simulink library "RxTxFixedPointLibrary_noscopes"  (R2020a)
settings: Solver=VariableStepAuto  StartTime=0.0  StopTime=10.0  RelTol=1e-3
undefined symbols (not defined in the file): AGCBarkerSymbols, coeff, crcDecodeLag, CRCGeneratorLag, EQTrainingSymbols, j, K1, K2, numHeaderBits, numTrainingSamples, pLen, RadioSampleRate, samplesPerSymbol, VibertiTracebackLength, xPreambleSeq
libraries: simulink x32, dsphdlfiltering x20, hdlsllib x13, commseqgen3 x4, dspsigops x4, commdigbbndpm3 x3, commcrc2 x2, commcnvcod2 x2, $bdroot x1, dspstat3 x1, commfilt2 x1
(part 2 of 3)

== system RxTxFixedPointLibrary_noscopes/Receiver HDL/Viterbi Decode/Subsystem ==
  BypassVit : Inport
  bitsIn : Inport  Port=2
  Reset : Inport  Port=3
  Demux : Demux  Outputs=2
  Switch : Switch  Criteria=u2 > Threshold
  Terminator : Terminator
  Viterbi Decoder : commcnvcod2/Viterbi Decoder  trellis=poly2trellis(7, [171 133])  isPunctured=off  punctureVector=[1; 1; 0; 1; 0; 1]  erasures=off  dectype=Hard decision  nsdecb=4  runSigValErrCheck=off  tbdepth=VibertiTracebackLength  opmode=Continuous  reset=on  delayedResetAction=on  smWordLength=16  outDataType=boolean
      settings: SourceProductBaseCode=CM
  Viterbi Lag2 : Delay  DelayLength=VibertiTracebackLength
  bitsOut : Outport  VectorParamsAs1DForOutWhenUnconnected=off
  wires:
  Switch/1 -> bitsOut/1
  Viterbi Decoder/1 -> Switch/3
  Demux/1 -> Viterbi Lag2/1
  Reset/1 -> Viterbi Decoder/2
  bitsIn/1 -> Demux/1, Viterbi Decoder/1
  BypassVit/1 -> Switch/2
  Demux/2 -> Terminator/1
  Viterbi Lag2/1 -> Switch/1

== system RxTxFixedPointLibrary_noscopes/Transmitter HDL/Packet Generation/Create Header ==
  In1 : Inport
  Duplicate Header Bits : Concatenate
  Logical Operator : Logic  Operator=NOT  Inputs=1  AllPortsSameDT=off  OutDataTypeStr=boolean
  Out1 : Outport  VectorParamsAs1DForOutWhenUnconnected=off
  wires:
  In1/1 -> Duplicate Header Bits/1, Logical Operator/1
  Duplicate Header Bits/1 -> Out1/1
  Logical Operator/1 -> Duplicate Header Bits/2

== system RxTxFixedPointLibrary_noscopes/Transmitter HDL/Packet Generation/Payload ==
  data : Inport
  start : Inport  Port=2
  done : Inport  Port=3
  BypassEncode : Inport  Port=4
  Allow Reset : Delay  DelayLength=1
  Allow Reset1 : Delay  DelayLength=1
  Compensate For Reset : Delay  DelayLength=1
  Compensate For Reset1 : Delay  DelayLength=1
  Convolutional Encoder : Subsystem
  General CRC Generator HDL Optimized : commcrc2/General CRC Generator HDL Optimized  Polynomial=[1 0 0 0 0 0 1 0 0 1 1 0 0 0 0 0 1 0 0 0 1 1 1 0 1 1 0 1 1 0 1 1 1]  InitialState=0  DirectMethod=off  ReflectInput=off  ReflectCRCChecksum=off  FinalXORValue=0  SimulateUsing=Code generation
      settings: SourceProductBaseCode=CM
  HDL Scrambler : Subsystem  mask{poly=[1 1 0 1 0 1 0 1], init_state=[0 1 0 0 0 1 0]}
      mask prompts: poly "Polynomial"; init_state "Initial State"
  Latch : Subsystem
  Switch : Switch  Criteria=u2 > Threshold
  Trackback Delay : Delay  DelayLength=VibertiTracebackLength*2
  Viterbi Lag Stuffer : Subsystem
  bits : Outport  VectorParamsAs1DForOutWhenUnconnected=off
  end : Outport  Port=2  VectorParamsAs1DForOutWhenUnconnected=off
  valid : Outport  Port=3  VectorParamsAs1DForOutWhenUnconnected=off
  wires:
  General CRC Generator HDL Optimized/1 -> Allow Reset/1
  General CRC Generator HDL Optimized/4 -> Compensate For Reset1/1
  General CRC Generator HDL Optimized/2 -> Convolutional Encoder/3(Reset), HDL Scrambler/2(reset)
  Convolutional Encoder/1(bitsOut) -> bits/1
  Compensate For Reset/1 -> Viterbi Lag Stuffer/1(EOF), Trackback Delay/1
  General CRC Generator HDL Optimized/3 -> Compensate For Reset/1
  Compensate For Reset1/1 -> valid/1
  Trackback Delay/1 -> end/1
  Latch/1(Out1) -> General CRC Generator HDL Optimized/4
  done/1 -> Latch/2(In2), General CRC Generator HDL Optimized/3
  Switch/1 -> Convolutional Encoder/2(bitsIn)
  BypassEncode/1 -> Convolutional Encoder/1(BypassEncode)
  data/1 -> General CRC Generator HDL Optimized/1
  start/1 -> Allow Reset1/1
  Allow Reset1/1 -> Latch/1(In1), General CRC Generator HDL Optimized/2
  Allow Reset/1 -> HDL Scrambler/1(bitsIn)
  HDL Scrambler/1(bitsOut) -> Switch/3
  Viterbi Lag Stuffer/1(Bits) -> Switch/1
  Viterbi Lag Stuffer/2(Mode) -> Switch/2

== system RxTxFixedPointLibrary_noscopes/Transmitter HDL/Packet Generation/Preamble ==
  reset : Inport
  Barker Even : LookupNDDirect  NumberOfTableDimensions=1  Table=[PreambleBarkersBits(4:2:end),false(1,400)]  DiagnosticForOutOfRangeInput=Error  TableDataTypeStr=boolean
  Barker Odd : LookupNDDirect  NumberOfTableDimensions=1  Table=[PreambleBarkersBits(3:2:end-1),false(1,400)]  DiagnosticForOutOfRangeInput=Error  TableDataTypeStr=boolean
  Delay{,1..3} (4 alike) : Delay  DelayLength=1
  Enable at end of barker : simulink/Logic and Bit Operations/Compare To Constant  relop=<  const=pLen/2-1  OutDataTypeStr=boolean
  HDL Counter : hdlsllib/Sources/HDL Counter  CountType=Count limited  CountInit=0  CountStep=1  CountMax=pLen/2-2+400  CountFromType=Initial value  CountFrom=0  CountResetPort=on  CountLoadPort=off  CountEnbPort=off  CountDirPort=off  CountDataType=Unsigned  CountWordLen=16  CountFracLen=0  CountSampTime=1
  PN Sequence For EQ : commseqgen3/PN Sequence Generator  poly='z^5 + z^3 + z^1 + 1'  ini_sta=[1 1 1 0 0]  outBitMaskSource=Dialog parameter  shift=0  outVarSiz=off  maxOutSizeMode=Dialog parameter  maxOutSize=[10 1]  Ts=-1  sampPerFrame=1  reset=on  bitPackedOutputs=on  outDataType=double  numPackedBits=2  bitPackDataSigned=off  bitPackedOutDType=Smallest integer
  Reset When Barkers Are Done : simulink/Logic and Bit Operations/Compare To Constant  relop===  const=pLen/2-1  OutDataTypeStr=boolean
  Switch1 : Switch  Threshold=1
  Unpack1 : Subsystem
  Vector Concatenate1 : Concatenate
  Out1 : Outport  VectorParamsAs1DForOutWhenUnconnected=off
  wires:
  reset/1 -> HDL Counter/1
  Barker Odd/1 -> Vector Concatenate1/1
  Barker Even/1 -> Vector Concatenate1/2
  PN Sequence For EQ/1 -> Unpack1/1(In1)
  Switch1/1 -> Out1/1
  Reset When Barkers Are Done/1 -> PN Sequence For EQ/1
  HDL Counter/1 -> Delay/1
  Delay/1 -> Enable at end of barker/1, Reset When Barkers Are Done/1, Barker Even/1, Barker Odd/1
  Vector Concatenate1/1 -> Delay1/1
  Enable at end of barker/1 -> Delay2/1
  Unpack1/1(Out1) -> Delay3/1
  Delay1/1 -> Switch1/1
  Delay2/1 -> Switch1/2
  Delay3/1 -> Switch1/3

== system RxTxFixedPointLibrary_noscopes/Transmitter HDL/Packet Generation/Random Data ==
  In1 : Inport
  Random Data Gen1 : commseqgen3/PN Sequence Generator  poly='z^10 + z^7 + 1'  ini_sta=[0 0 1 0 0 1 0 0 1 1]  outBitMaskSource=Dialog parameter  shift=0  outVarSiz=off  maxOutSizeMode=Dialog parameter  maxOutSize=[10 1]  Ts=-1  sampPerFrame=1  reset=on  bitPackedOutputs=on  outDataType=double  numPackedBits=2  bitPackDataSigned=off  bitPackedOutDType=Smallest integer
  Unpack : Subsystem
  Out1 : Outport  VectorParamsAs1DForOutWhenUnconnected=off
  wires:
  In1/1 -> Random Data Gen1/1
  Unpack/1(Out1) -> Out1/1
  Random Data Gen1/1 -> Unpack/1(In1)

== system RxTxFixedPointLibrary_noscopes/Receiver HDL/CRC Check and DMA Pack/DMA Interface/Convert Payload Length To Bytes ==
  In1 : Inport
  Constant : Constant  Value=uint16(32-1)  SampleTime=-1
  Convert To Bytes From Bits : ArithShift  BitShiftNumber=3  BitShiftDirection=Right
  Convert To Uncoded : ArithShift  BitShiftNumber=1  BitShiftDirection=Right
  Data Type Conversion : DataTypeConversion  OutDataTypeStr=uint16
  Remove CRC Length : Sum  Inputs=+-  AccumDataTypeStr=uint16
  packetLengthOut : Outport  VectorParamsAs1DForOutWhenUnconnected=off
  wires:
  Data Type Conversion/1 -> packetLengthOut/1
  Constant/1 -> Remove CRC Length/2
  Convert To Bytes From Bits/1 -> Data Type Conversion/1
  Convert To Uncoded/1 -> Remove CRC Length/1
  Remove CRC Length/1 -> Convert To Bytes From Bits/1
  In1/1 -> Convert To Uncoded/1

== system RxTxFixedPointLibrary_noscopes/Receiver HDL/Frame Recover/Barker Locate/ABS1 ==
  In1 : Inport
  Add : Sum
  Complex to Real-Imag : ComplexToRealImag
  Product : Product  OutDataTypeStr=int16
  Product1 : Product  OutDataTypeStr=int16
  Out1 : Outport  VectorParamsAs1DForOutWhenUnconnected=off
  wires:
  Add/1 -> Out1/1
  Product1/1 -> Add/2
  Product/1 -> Add/1
  Complex to Real-Imag/1 -> Product/2, Product/1
  Complex to Real-Imag/2 -> Product1/1, Product1/2
  In1/1 -> Complex to Real-Imag/1

== system RxTxFixedPointLibrary_noscopes/Receiver HDL/Frame Recover/Barker Locate/ABS2 ==
  In1 : Inport
  Add : Sum  SaturateOnIntegerOverflow=on
  Complex to Real-Imag : ComplexToRealImag
  Product : Product  OutDataTypeStr=int16
  Product1 : Product  OutDataTypeStr=int16
  Out1 : Outport  VectorParamsAs1DForOutWhenUnconnected=off
  wires:
  Add/1 -> Out1/1
  Product1/1 -> Add/2
  Product/1 -> Add/1
  Complex to Real-Imag/1 -> Product/2, Product/1
  Complex to Real-Imag/2 -> Product1/1, Product1/2
  In1/1 -> Complex to Real-Imag/1

== system RxTxFixedPointLibrary_noscopes/Receiver HDL/Frame Recover/Barker Locate/HDL Opt Complex FIR ==
  In1 : Inport
  validIn : Inport  Port=2
  Add : Sum  AccumDataTypeStr=fixdt(1,16,0)
  Constant : Constant  Value=real(Taps)  OutDataTypeStr=fixdt(1,16)  SampleTime=-1
  Constant1 : Constant  Value=imag(Taps)  OutDataTypeStr=fixdt(1,16)  SampleTime=-1
  Discrete FIR Filter HDL Optimized : dsphdlfiltering/Discrete FIR Filter HDL Optimized  NumeratorSource=Input port (Parallel interface)  Numerator=real(Taps)  NumeratorPrototype=[]  FilterStructure=Direct form systolic  SerializationOption=Minimum number of cycles between valid input samples  NumberOfCycles=2  NumberOfMultipliers=2  SimulateUsing=Code generation  roundingMode=Floor  overflowMode=off  CoefficientsDataTypeStr=Inherit: Same word length as input  CoefficientsMin=[]  CoefficientsMax=[]  OutputDataTypeStr=fixdt(1,15,0)  OutputMin=[]  OutputMax=[]  ResetInputPort=off  HDLGlobalReset=off
      settings: SourceProductBaseCode=DS
  Discrete FIR Filter HDL Optimized1 : dsphdlfiltering/Discrete FIR Filter HDL Optimized  NumeratorSource=Input port (Parallel interface)  Numerator=imag(Taps)  NumeratorPrototype=[]  FilterStructure=Direct form systolic  SerializationOption=Minimum number of cycles between valid input samples  NumberOfCycles=2  NumberOfMultipliers=2  SimulateUsing=Code generation  roundingMode=Floor  overflowMode=off  CoefficientsDataTypeStr=Inherit: Same word length as input  CoefficientsMin=[]  CoefficientsMax=[]  OutputDataTypeStr=fixdt(1,15,0)  OutputMin=[]  OutputMax=[]  ResetInputPort=off  HDLGlobalReset=off
      settings: SourceProductBaseCode=DS
  Logical Operator : Logic  AllPortsSameDT=off  OutDataTypeStr=boolean
  Out1 : Outport  VectorParamsAs1DForOutWhenUnconnected=off
  validOut : Outport  Port=2  VectorParamsAs1DForOutWhenUnconnected=off
  wires:
  Constant1/1 -> Discrete FIR Filter HDL Optimized1/3
  Constant/1 -> Discrete FIR Filter HDL Optimized/3
  validIn/1 -> Discrete FIR Filter HDL Optimized/2, Discrete FIR Filter HDL Optimized1/2
  Discrete FIR Filter HDL Optimized1/1 -> Add/2
  Discrete FIR Filter HDL Optimized1/2 -> Logical Operator/2
  Discrete FIR Filter HDL Optimized/2 -> Logical Operator/1
  Logical Operator/1 -> validOut/1
  Add/1 -> Out1/1
  Discrete FIR Filter HDL Optimized/1 -> Add/1
  In1/1 -> Discrete FIR Filter HDL Optimized/1, Discrete FIR Filter HDL Optimized1/1

== system RxTxFixedPointLibrary_noscopes/Receiver HDL/Frame Recover/Barker Locate/Measure Phase Ambiguity ==
  data : Inport  OutDataTypeStr=int16
  trigger : Inport  Port=2
  validIn : Inport  Port=3
  Delay{,1..3} (4 alike) : Delay  DelayLength=1
  Find Max and Set Output Shift : Subsystem
  HDL Opt Complex FIR4 : Subsystem  mask{Taps=xPreambleSeq(end:-1:1).'}
  HDL Opt Complex FIR5 : Subsystem  mask{Taps=exp(-j*pi/2).*xPreambleSeq(end:-1:1).'}
  HDL Opt Complex FIR6 : Subsystem  mask{Taps=exp(-j*pi).*xPreambleSeq(end:-1:1).'}
  HDL Opt Complex FIR7 : Subsystem  mask{Taps=exp(-j*pi*3/2).*xPreambleSeq(end:-1:1).'}
  Logical Operator : Logic  Inputs=5  AllPortsSameDT=off  OutDataTypeStr=boolean
  Terminator : Terminator
  PA : Outport  InitialOutput=0  VectorParamsAs1DForOutWhenUnconnected=off
  wires:
  Logical Operator/1 -> Terminator/1
  Delay3/1 -> Find Max and Set Output Shift/1(In1)
  Delay2/1 -> Find Max and Set Output Shift/2(In2)
  Delay1/1 -> Find Max and Set Output Shift/3(In4)
  Delay/1 -> Find Max and Set Output Shift/4(In5)
  trigger/1 -> Logical Operator/5, Find Max and Set Output Shift/Enable
  HDL Opt Complex FIR7/2(validOut) -> Logical Operator/4
  HDL Opt Complex FIR6/2(validOut) -> Logical Operator/3
  HDL Opt Complex FIR5/2(validOut) -> Logical Operator/2
  HDL Opt Complex FIR4/2(validOut) -> Logical Operator/1
  validIn/1 -> HDL Opt Complex FIR6/2(validIn), HDL Opt Complex FIR7/2(validIn), HDL Opt Complex FIR5/2(validIn), HDL Opt Complex FIR4/2(validIn)
  Find Max and Set Output Shift/1(Out1) -> PA/1
  HDL Opt Complex FIR7/1(Out1) -> Delay/1
  HDL Opt Complex FIR6/1(Out1) -> Delay1/1
  HDL Opt Complex FIR5/1(Out1) -> Delay2/1
  HDL Opt Complex FIR4/1(Out1) -> Delay3/1
  data/1 -> HDL Opt Complex FIR6/1(In1), HDL Opt Complex FIR7/1(In1), HDL Opt Complex FIR5/1(In1), HDL Opt Complex FIR4/1(In1)

== system RxTxFixedPointLibrary_noscopes/Receiver HDL/Frame Recover/Equalization and Demodulation/DFE ==
  note: Generate training sequence when barker is found
  note: refTap=0 to disableEQ
  Trigger : Inport  PortDimensions=1
  data : Inport  Port=2  PortDimensions=1
      settings: SignalType=complex
  EQmu : Inport  Port=3
  eqBypass : Inport  Port=4
  DFE : Subsystem  mask{numFTaps=5, numBTaps=3, mu=0.01, refTap=2}
      mask prompts: numFTaps "Num Forward Taps"; numBTaps "Num Backward Taps"; mu "Step Size"; refTap "Reference Tap"
  Delay data so DFE can reset : Delay  DelayLength=1
  Delay ref so DFE can reset : Delay  DelayLength=1
  Equalizer : MATLAB Function  Commented=on  TreatAsAtomicUnit=on
  PN Sequence Generator : commseqgen3/PN Sequence Generator  poly='z^5 + z^3 + z^1 + 1'  ini_sta=[1 1 1 0 0]  outBitMaskSource=Dialog parameter  shift=0  outVarSiz=off  maxOutSizeMode=Dialog parameter  maxOutSize=[10 1]  Ts=-1  sampPerFrame=1  reset=on  bitPackedOutputs=on  outDataType=Smallest unsigned integer  numPackedBits=2  bitPackDataSigned=off  bitPackedOutDType=Smallest integer
  Packeted To Unpacked : Subsystem
  QPSK Modulator Baseband : commdigbbndpm3/QPSK Modulator Baseband  InType=Bit  Enc=Binary  Ph=pi/4  outDtype=Fixed-point  outWordLen=16  outUDDataType=sfix(16)  outFracLenMode=User-defined  outFracLen=15  outDataTypeStr=fixdt(1,16,15)  outLastDataTypeStr=fixdt(1,16,15)
  Terminator1 : Terminator
  dataEQed : Outport  VectorParamsAs1DForOutWhenUnconnected=off
  start : Outport  Port=2  VectorParamsAs1DForOutWhenUnconnected=off
  wires:
  EQmu/1 -> DFE/4(EQmu)
  Delay ref so DFE can reset/1 -> DFE/3(training)
  Delay data so DFE can reset/1 -> DFE/2(dataIn)
  DFE/1(eqOut) -> dataEQed/1
  DFE/2(err) -> Terminator1/1
  Trigger/1 -> PN Sequence Generator/1, DFE/1(reset)
  DFE/3(start) -> start/1
  QPSK Modulator Baseband/1 -> Delay ref so DFE can reset/1
  Packeted To Unpacked/1(Out1) -> QPSK Modulator Baseband/1
  PN Sequence Generator/1 -> Packeted To Unpacked/1(In1)
  data/1 -> Delay data so DFE can reset/1
  eqBypass/1 -> DFE/5(eqBypass)

== system RxTxFixedPointLibrary_noscopes/Receiver HDL/Frame Recover/Frequency Recovery/Lock Detector ==
  ped : Inport
  Compare To Constant : simulink/Logic and Bit Operations/Compare To Constant  relop=<=  const=Threshold*WindowLength  OutDataTypeStr=boolean
  MATLAB Function : MATLAB Function  TreatAsAtomicUnit=on
  Pipeline Delay{,1..3} (4 alike) : Delay  DelayLength=1
  Sum of Elements : Sum  Inputs=+
  Tapped Delay : simulink/Discrete/Tapped Delay  vinit=0.0  samptime=-1  NumDelays=WindowLength  DelayOrder=Oldest  includeCurrent=off
  lock : Outport  VectorParamsAs1DForOutWhenUnconnected=off
  wires:
  ped/1 -> Pipeline Delay/1
  Tapped Delay/1 -> Pipeline Delay2/1
  Sum of Elements/1 -> Pipeline Delay3/1
  Compare To Constant/1 -> lock/1
  MATLAB Function/1(y) -> Pipeline Delay1/1
  Pipeline Delay/1 -> MATLAB Function/1(u)
  Pipeline Delay1/1 -> Tapped Delay/1
  Pipeline Delay2/1 -> Sum of Elements/1
  Pipeline Delay3/1 -> Compare To Constant/1

== system RxTxFixedPointLibrary_noscopes/Receiver HDL/Frame Recover/Frequency Recovery/Loop Filter ==
  note: Proportional-plus-Integrator Loop Filter,
      | Infinite DC Response to guarantee convergence
  note: This inflation is necessary
  e : Inport
  Add1 : Sum  RndMeth=Nearest  OutDataTypeStr=Inherit: Same as first input
  Add2 : Sum  OutDataTypeStr=Inherit: Same as first input
  Data Type Conversion : DataTypeConversion  OutDataTypeStr=fixdt(1,25,20)
  Delay : Delay  DelayLength=1
  Delay3 : Delay  DelayLength=1
  Delay4 : Delay  DelayLength=1
  K1 : Gain  Gain=K2  OutDataTypeStr=Inherit: Same as input
  K2 : Gain  Gain=K1  OutDataTypeStr=Inherit: Same as input
  Sum2 : Sum  OutDataTypeStr=Inherit: Same as first input
  v : Outport  VectorParamsAs1DForOutWhenUnconnected=off
  wires:
  Data Type Conversion/1 -> v/1
  Add2/1 -> Data Type Conversion/1, Delay4/1
  Delay4/1 -> Add2/2
  Delay3/1 -> Add2/1
  Sum2/1 -> Delay3/1
  Delay/1 -> Add1/1
  K2/1 -> Add1/2, Delay/1
  e/1 -> K1/1, K2/1
  Add1/1 -> Sum2/2
  K1/1 -> Sum2/1

== system RxTxFixedPointLibrary_noscopes/Receiver HDL/Frame Recover/Frequency Recovery/Loop Filter Configurable ==
  note: Proportional-plus-Integrator Loop Filter,
      | Infinite DC Response to guarantee convergence
  note: This inflation is necessary
  e : Inport
  LoopBW : Inport  Port=2
  Add1 : Sum  RndMeth=Nearest  OutDataTypeStr=Inherit: Same as first input
  Add2 : Sum  OutDataTypeStr=Inherit: Same as first input
  Data Type Conversion : DataTypeConversion  OutDataTypeStr=fixdt(1,25,20)
  Delay : Delay  DelayLength=1
  Delay3 : Delay  DelayLength=1
  Delay4 : Delay  DelayLength=1
  Direct Lookup Table (n-D) : LookupNDDirect  NumberOfTableDimensions=1  Table=K1  DiagnosticForOutOfRangeInput=Error
  Direct Lookup Table (n-D)1 : LookupNDDirect  NumberOfTableDimensions=1  Table=K2  DiagnosticForOutOfRangeInput=Error
  Product : Product  OutDataTypeStr=Inherit: Same as first input
  Product1 : Product  OutDataTypeStr=Inherit: Same as first input
  Sum2 : Sum  OutDataTypeStr=Inherit: Same as first input
  v : Outport  VectorParamsAs1DForOutWhenUnconnected=off
  wires:
  LoopBW/1 -> Direct Lookup Table (n-D)1/1, Direct Lookup Table (n-D)/1
  Direct Lookup Table (n-D)1/1 -> Product1/2
  Direct Lookup Table (n-D)/1 -> Product/2
  Data Type Conversion/1 -> v/1
  Add2/1 -> Data Type Conversion/1, Delay4/1
  Delay4/1 -> Add2/2
  Delay3/1 -> Add2/1
  Sum2/1 -> Delay3/1
  Delay/1 -> Add1/1
  Product1/1 -> Add1/2, Delay/1
  e/1 -> Product/1, Product1/1
  Add1/1 -> Sum2/2
  Product/1 -> Sum2/1

== system RxTxFixedPointLibrary_noscopes/Receiver HDL/Frame Recover/Frequency Recovery/Phase Shift FP ==
  note: Sign Comes from original
      | loop filter design
  In1 : Inport
  Phi : Inport  Port=2
  Cosine HDL Optimized : hdlsllib/Lookup Tables/Cosine HDL Optimized  OutputFormula=exp(j*2*pi*u)  NumDataPoints=256  TableDataTypeStr=fixdt(0,31,20)  SimulateLUTROMDelay=off
      settings: SourceProductBaseCode=SL
  Gain : Gain  Gain=-1/(2*pi)  ParamDataTypeStr=fixdt(1,25,20)  OutDataTypeStr=fixdt(1,16,12)  SaturateOnIntegerOverflow=on
  Product : Product  OutDataTypeStr=fixdt(1,16,13)  SaturateOnIntegerOverflow=on
  Out1 : Outport  VectorParamsAs1DForOutWhenUnconnected=off
  wires:
  Gain/1 -> Cosine HDL Optimized/1
  Phi/1 -> Gain/1
  In1/1 -> Product/1
  Cosine HDL Optimized/1 -> Product/2
  Product/1 -> Out1/1

== system RxTxFixedPointLibrary_noscopes/Receiver HDL/Frame Recover/Gardner Timing Recovery/Gardner TED Blocks ==
  note: This is for QPSK and 4 SamplesPerSymbol ONLY
  note: An input of 4 should not
      | happen unless the input is all zeros
  data : Inport
  strobe : Inport  Port=2
  Add : Sum  OutDataTypeStr=fixdt(1,16,15)
  Check Only Strobe Condition : simulink/Logic and Bit Operations/Compare To Constant  relop===  const=uint8(1)  OutDataTypeStr=boolean
  Complex to Real-Imag : ComplexToRealImag
  Constant : Constant  Value=0  OutDataTypeStr=Inherit: Inherit via back propagation  SampleTime=-1
  Display : Display
  Imag Error : Subsystem
  Logical Operator : Logic  AllPortsSameDT=off  OutDataTypeStr=boolean
  Map [0,1,2,3,4] to [0,1,2,2,2] : LookupNDDirect  NumberOfTableDimensions=1  Table=[0 1 2 2 2]  DiagnosticForOutOfRangeInput=Error  TableDataTypeStr=uint8
  Real Error : Subsystem
  Strobe Buffer1 : simulink/Discrete/Tapped Delay  vinit=0.0  samptime=-1  NumDelays=samplesPerSymbol-1  DelayOrder=Oldest  includeCurrent=on
  Sum of Elements1 : Sum  Inputs=+  OutDataTypeStr=int8
  Switch : Switch  Criteria=u2 ~= 0  SaturateOnIntegerOverflow=on
  e : Outport  VectorParamsAs1DForOutWhenUnconnected=off
  wires:
  Logical Operator/1 -> Switch/2
  Add/1 -> Switch/1
  Imag Error/1(Out1) -> Add/2
  Real Error/1(Out1) -> Add/1
  Strobe Buffer1/1 -> Sum of Elements1/1
  Map [0,1,2,3,4] to [0,1,2,2,2]/1 -> Real Error/2(strobe sum), Imag Error/2(strobe sum)
  data/1 -> Complex to Real-Imag/1
  Complex to Real-Imag/1 -> Real Error/1(data)
  Constant/1 -> Switch/3
  Check Only Strobe Condition/1 -> Logical Operator/1
  Sum of Elements1/1 -> Map [0,1,2,3,4] to [0,1,2,2,2]/1, Check Only Strobe Condition/1, Display/1
  Complex to Real-Imag/2 -> Imag Error/1(data)
  strobe/1 -> Logical Operator/2, Strobe Buffer1/1
  Switch/1 -> e/1

== system RxTxFixedPointLibrary_noscopes/Receiver HDL/Frame Recover/Gardner Timing Recovery/InterpControl_Blocks1 ==
  note: Mu is always positive
  note: e<<1/SPS
  e : Inport
  1/SPS1 : Constant  Value=fi(1/samplesPerSymbol,0,2,2)  OutDataTypeStr=fixdt(0,2,2)  SampleTime=-1
  Add1 : Sum  OutDataTypeStr=fixdt(0,16,16)
  Calculate New mu : Subsystem
  Display{,1..3} (4 alike) : Display
  Mod 1 : Subsystem
  NCOCounter State : Delay  DelayLength=1  InitialCondition=0
  Subtract1 : Sum  Inputs=-+  OutDataTypeStr=Inherit: Same as first input
  Update mu on strobe : Switch  Criteria=u2 > Threshold
  saved mu : Delay  DelayLength=1
  strobe == W>NCOCounter : RelationalOperator  Operator=>  OutDataTypeStr=boolean  RndMeth=Nearest
  strobe : Outport  VectorParamsAs1DForOutWhenUnconnected=off
  mu : Outport  Port=2  VectorParamsAs1DForOutWhenUnconnected=off
  wires:
  Add1/1 -> Subtract1/1, Display2/1, strobe == W>NCOCounter/1, Calculate New mu/1(W)
  1/SPS1/1 -> Add1/2
  Mod 1/1(Out1) -> NCOCounter State/1
  Subtract1/1 -> Mod 1/1(In1)
  NCOCounter State/1 -> Calculate New mu/2(NCOCounter), strobe == W>NCOCounter/2, Display1/1, Subtract1/2
  e/1 -> Add1/1
  Calculate New mu/1(mu) -> Update mu on strobe/1, Display/1
  saved mu/1 -> Update mu on strobe/3
  Update mu on strobe/1 -> saved mu/1, mu/1, Display3/1
  strobe == W>NCOCounter/1 -> strobe/1, Update mu on strobe/2

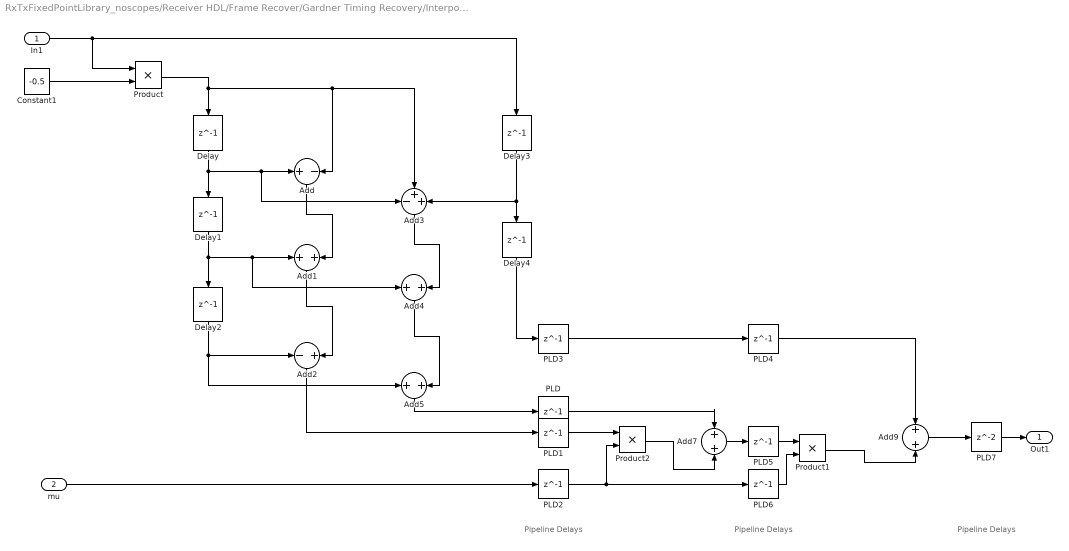
== system RxTxFixedPointLibrary_noscopes/Receiver HDL/Frame Recover/Gardner Timing Recovery/Interpolator ==
  note: Pipeline Delays
  note: Pipeline Delays
  note: Pipeline Delays
  In1 : Inport
  mu : Inport  Port=2
  Add : Sum  Inputs=+-  OutDataTypeStr=Inherit: Same as first input
  Add{1,4..5,7} (4 alike) : Sum
  Add2 : Sum  Inputs=-+
  Add3 : Sum  Inputs=-++
  Add9 : Sum  OutDataTypeStr=fixdt(1,16,10)
  Constant1 : Constant  Value=-0.5  OutDataTypeStr=fixdt(1,2,2)  SampleTime=-1
  Delay{,1..4} (5 alike) : Delay  DelayLength=1
  PLD{,1..6} (7 alike) : Delay  DelayLength=1
  PLD7 : Delay
  Product : Product  OutDataTypeStr=fixdt(1,16,14)
  Product1 : Product
  Product2 : Product  OutDataTypeStr=fixdt(1,16,10)
  Out1 : Outport  VectorParamsAs1DForOutWhenUnconnected=off
  wires:
  PLD7/1 -> Out1/1
  PLD6/1 -> Product1/2
  PLD5/1 -> Product1/1
  PLD4/1 -> Add9/1
  PLD3/1 -> PLD4/1
  PLD2/1 -> PLD6/1, Product2/2
  PLD1/1 -> Product2/1
  PLD/1 -> Add7/1
  Constant1/1 -> Product/2
  Product1/1 -> Add9/2
  Add7/1 -> PLD5/1
  Delay4/1 -> PLD3/1
  Delay3/1 -> Add3/3, Delay4/1
  Add9/1 -> PLD7/1
  Product2/1 -> Add7/2
  Add5/1 -> PLD/1
  mu/1 -> PLD2/1
  Add2/1 -> PLD1/1
  Add4/1 -> Add5/2
  Add3/1 -> Add4/2
  Add1/1 -> Add2/2
  Delay2/1 -> Add2/1, Add5/1
  Add/1 -> Add1/2
  Delay1/1 -> Delay2/1, Add1/1, Add4/1
  Delay/1 -> Delay1/1, Add/1, Add3/1
  Product/1 -> Delay/1, Add/2, Add3/2
  In1/1 -> Product/1, Delay3/1

== system RxTxFixedPointLibrary_noscopes/Receiver HDL/Frame Recover/Gardner Timing Recovery/LoopFilter1 ==
  e : Inport
  Delay1 : Delay  DelayLength=1
  Delay2 : Delay  DelayLength=1
  Proportional Gain : Gain  Gain=fi(ProportionalGain,1,16,15)  OutDataTypeStr=fixdt(1,16,24)
  v : Outport  VectorParamsAs1DForOutWhenUnconnected=off
  wires:
  Delay1/1 -> v/1
  Delay2/1 -> Proportional Gain/1
  Proportional Gain/1 -> Delay1/1
  e/1 -> Delay2/1

== system RxTxFixedPointLibrary_noscopes/Receiver HDL/Frame Recover/Gardner Timing Recovery/TED Lock Detector ==
  ted : Inport
  Compare To Constant : simulink/Logic and Bit Operations/Compare To Constant  relop=<=  const=Threshold*WindowLength  OutDataTypeStr=boolean
  MATLAB Function : MATLAB Function  TreatAsAtomicUnit=on
  Pipeline Delay{,1..3} (4 alike) : Delay  DelayLength=1
  Sum of Elements : Sum  Inputs=+
  Tapped Delay : simulink/Discrete/Tapped Delay  vinit=0.0  samptime=-1  NumDelays=WindowLength  DelayOrder=Oldest  includeCurrent=off
  lock : Outport  VectorParamsAs1DForOutWhenUnconnected=off
  wires:
  ted/1 -> Pipeline Delay/1
  Tapped Delay/1 -> Pipeline Delay1/1
  Sum of Elements/1 -> Pipeline Delay3/1
  Compare To Constant/1 -> lock/1
  MATLAB Function/1(y) -> Pipeline Delay2/1
  Pipeline Delay/1 -> MATLAB Function/1(u)
  Pipeline Delay1/1 -> Sum of Elements/1
  Pipeline Delay2/1 -> Tapped Delay/1
  Pipeline Delay3/1 -> Compare To Constant/1

== system RxTxFixedPointLibrary_noscopes/Receiver HDL/Frame Recover/Manage Error Signals/Debug: Header Check ==
  <status> : Inport
  <s1> : Inport  Port=2
  <s2> : Inport  Port=3
  Enable : EnablePort
  DEBUG: Header : MATLAB Function  TreatAsAtomicUnit=on
  wires:
  <s1>/1 -> DEBUG: Header/2(h1)
  <status>/1 -> DEBUG: Header/1(status)
  <s2>/1 -> DEBUG: Header/3(h2)

== system RxTxFixedPointLibrary_noscopes/Receiver HDL/Viterbi Decode/Buffer Frame/Check Packet Size ==
  In1 : Inport
  In2 : Inport  Port=2
  In3 : Inport  Port=3
  Compare To Zero : simulink/Logic and Bit Operations/Compare To Zero  relop=~=  OutDataTypeStr=boolean
  HDL Counter1 : hdlsllib/Sources/HDL Counter  CountType=Count limited  CountInit=0  CountStep=1  CountMax=2^16-1  CountFromType=Initial value  CountFrom=0  CountResetPort=off  CountLoadPort=off  CountEnbPort=on  CountDirPort=off  CountDataType=Unsigned  CountWordLen=16  CountFracLen=0  CountSampTime=1
  Logical Operator1 : Logic  AllPortsSameDT=off  OutDataTypeStr=boolean
  Pipeline Delay{,1..3} (4 alike) : Delay  DelayLength=1
  Subtract1 : Sum  Inputs=+-
  Out1 : Outport  VectorParamsAs1DForOutWhenUnconnected=off
  wires:
  Pipeline Delay3/1 -> Out1/1
  Pipeline Delay2/1 -> Logical Operator1/2
  Pipeline Delay1/1 -> Subtract1/2
  Pipeline Delay/1 -> Subtract1/1
  In3/1 -> Pipeline Delay2/1
  HDL Counter1/1 -> Pipeline Delay3/1
  In1/1 -> Pipeline Delay/1
  In2/1 -> Pipeline Delay1/1
  Logical Operator1/1 -> HDL Counter1/1
  Compare To Zero/1 -> Logical Operator1/1
  Subtract1/1 -> Compare To Zero/1

== system RxTxFixedPointLibrary_noscopes/Receiver HDL/Viterbi Decode/Buffer Frame/FIFO ==
  dataIn : Inport
  Push : Inport  Port=2
  Pop : Inport  Port=3
  Demux : Demux  Outputs=2
  HDL FIFO3 : hdlsllib/HDL RAMs/HDL FIFO  fifo_size=2^16  mode=Classic  ratio=1  push_msg=Warning  pop_msg=Warning  show_empty=off  show_full=off  show_num=on  LabelModeActiveChoice_Mode=Classic
      settings: SourceProductBaseCode=SL
  HDL FIFO4 : hdlsllib/HDL RAMs/HDL FIFO  fifo_size=2^16  mode=Classic  ratio=1  push_msg=Warning  pop_msg=Warning  show_empty=off  show_full=off  show_num=off  LabelModeActiveChoice_Mode=Classic
      settings: SourceProductBaseCode=SL
  Mux : Mux  Inputs=2
  dataOut : Outport  VectorParamsAs1DForOutWhenUnconnected=off
  Count : Outport  Port=2  VectorParamsAs1DForOutWhenUnconnected=off
  wires:
  HDL FIFO3/2 -> Count/1
  HDL FIFO4/1 -> Mux/2
  Mux/1 -> dataOut/1
  HDL FIFO3/1 -> Mux/1
  Demux/2 -> HDL FIFO4/1
  Demux/1 -> HDL FIFO3/1
  dataIn/1 -> Demux/1
  Push/1 -> HDL FIFO3/2, HDL FIFO4/2
  Pop/1 -> HDL FIFO3/3, HDL FIFO4/3

== system RxTxFixedPointLibrary_noscopes/Receiver HDL/Viterbi Decode/Buffer Frame/Latch ==
  In1 : Inport
  In2 : Inport  Port=2
  Delay2 : Delay  DelayLength=1
  Switch : Switch  Criteria=u2 > Threshold  OutDataTypeStr=fixdt(0,17,0)
  Out1 : Outport  VectorParamsAs1DForOutWhenUnconnected=off
  wires:
  Switch/1 -> Delay2/1, Out1/1
  Delay2/1 -> Switch/3
  In1/1 -> Switch/1
  In2/1 -> Switch/2

== system RxTxFixedPointLibrary_noscopes/Receiver HDL/Viterbi Decode/Descrambler1/Resetabled Tapped Delay ==
  In1 : Inport
  Reset : ResetPort  DisableCoverage=on  ResetTriggerType=level hold
  State Control : StateControl  StateControl=Synchronous
  Tapped Delay : simulink/Discrete/Tapped Delay  vinit=initstate(1:end)  samptime=-1  NumDelays=length(initstate)  DelayOrder=Oldest  includeCurrent=off
  Out1 : Outport  VectorParamsAs1DForOutWhenUnconnected=off
  wires:
  In1/1 -> Tapped Delay/1
  Tapped Delay/1 -> Out1/1

== system RxTxFixedPointLibrary_noscopes/Transmitter HDL/Packet Generation/Payload/Convolutional Encoder ==
  BypassEncode : Inport
  bitsIn : Inport  Port=2
  Reset : Inport  Port=3
  Convolutional Encoder : commcnvcod2/Convolutional Encoder  trellis=poly2trellis(7, [171 133])  opMode=Reset on nonzero input via port  DelayedResetAction=on  hasIniStPort=off  hasFinStPort=off  usePuncVector=off  punctureVector=[1; 1; 0; 1; 0; 1]  reset=Unused parameter value
      settings: SourceProductBaseCode=CM
  Mux : Mux  Inputs=2
  Signal Specification : SignalSpecification  Dimensions=2
  Switch1 : Switch  Criteria=u2 > Threshold
  bitsOut : Outport  VectorParamsAs1DForOutWhenUnconnected=off
  wires:
  bitsIn/1 -> Mux/2, Mux/1, Convolutional Encoder/1
  Mux/1 -> Switch1/1
  Reset/1 -> Convolutional Encoder/2
  BypassEncode/1 -> Switch1/2
  Switch1/1 -> bitsOut/1
  Convolutional Encoder/1 -> Signal Specification/1
  Signal Specification/1 -> Switch1/3

== system RxTxFixedPointLibrary_noscopes/Transmitter HDL/Packet Generation/Payload/HDL Scrambler ==
  bitsIn : Inport
  reset : Inport  Port=2
  Resettable Synchronous Subsystem : Subsystem  TreatAsAtomicUnit=on
  Selector2 : Selector  IndexOptions=Index vector (dialog)  Indices=find(poly(2:end))  OutputSizes=1
  state_xor5 : Logic  Operator=XOR  Inputs=1  IconShape=distinctive  AllPortsSameDT=off  OutDataTypeStr=boolean
  state_xor6 : Logic  Operator=XOR  IconShape=distinctive  AllPortsSameDT=off  OutDataTypeStr=boolean
  bitsOut : Outport  VectorParamsAs1DForOutWhenUnconnected=off
  wires:
  reset/1 -> Resettable Synchronous Subsystem/Reset
  Selector2/1 -> state_xor5/1
  state_xor5/1 -> state_xor6/1
  bitsIn/1 -> state_xor6/2
  Resettable Synchronous Subsystem/1(Out1) -> Selector2/1
  state_xor6/1 -> Resettable Synchronous Subsystem/1(In1), bitsOut/1

== system RxTxFixedPointLibrary_noscopes/Transmitter HDL/Packet Generation/Payload/Latch ==
  In1 : Inport
  In2 : Inport  Port=2
  Logical Operator : Logic  Operator=OR  Inputs=3  AllPortsSameDT=off  OutDataTypeStr=boolean
  MATLAB Function3 : MATLAB Function  TreatAsAtomicUnit=on
  Out1 : Outport  VectorParamsAs1DForOutWhenUnconnected=off
  wires:
  In2/1 -> Logical Operator/3, MATLAB Function3/2(done)
  In1/1 -> Logical Operator/1, MATLAB Function3/1(start)
  MATLAB Function3/1(enable) -> Logical Operator/2
  Logical Operator/1 -> Out1/1

== system RxTxFixedPointLibrary_noscopes/Transmitter HDL/Packet Generation/Payload/Viterbi Lag Stuffer ==
  EOF : Inport
  Compensate For Data2 : Delay  DelayLength=1
  MATLAB Function : MATLAB Function  TreatAsAtomicUnit=on
  Random Data Gen1 : commseqgen3/PN Sequence Generator  poly='z^10 + z^7 + 1'  ini_sta=[0 0 1 0 0 1 0 0 1 1]  outBitMaskSource=Dialog parameter  shift=0  outVarSiz=off  maxOutSizeMode=Dialog parameter  maxOutSize=[10 1]  Ts=-1  sampPerFrame=1  reset=on  bitPackedOutputs=on  outDataType=double  numPackedBits=1  bitPackDataSigned=off  bitPackedOutDType=Smallest integer
  Bits : Outport  VectorParamsAs1DForOutWhenUnconnected=off
  Mode : Outport  Port=2  VectorParamsAs1DForOutWhenUnconnected=off
  wires:
  MATLAB Function/2(mode) -> Mode/1
  MATLAB Function/1(reset) -> Random Data Gen1/1
  Random Data Gen1/1 -> Bits/1
  Compensate For Data2/1 -> MATLAB Function/1(enable)
  EOF/1 -> Compensate For Data2/1

== system RxTxFixedPointLibrary_noscopes/Transmitter HDL/Packet Generation/Preamble/Unpack1 ==
  In1 : Inport
  Data Type Conversion : DataTypeConversion  OutDataTypeStr=boolean
  Extract Bits : simulink/Logic and Bit Operations/Extract Bits  bitsToExtract=Range of bits  numBits=8  bitIdxRange=[1]  outScalingMode=Treat bit field as an integer
  Extract Bits1 : simulink/Logic and Bit Operations/Extract Bits  bitsToExtract=Range of bits  numBits=8  bitIdxRange=[0]  outScalingMode=Treat bit field as an integer
  Vector Concatenate : Concatenate
  Out1 : Outport  VectorParamsAs1DForOutWhenUnconnected=off
  wires:
  In1/1 -> Extract Bits1/1, Extract Bits/1
  Extract Bits/1 -> Vector Concatenate/1
  Extract Bits1/1 -> Vector Concatenate/2
  Vector Concatenate/1 -> Data Type Conversion/1
  Data Type Conversion/1 -> Out1/1

== system RxTxFixedPointLibrary_noscopes/Transmitter HDL/Packet Generation/Random Data/Unpack ==
  In1 : Inport
  Data Type Conversion : DataTypeConversion  OutDataTypeStr=boolean
  Extract Bits : simulink/Logic and Bit Operations/Extract Bits  bitsToExtract=Range of bits  numBits=8  bitIdxRange=[0]  outScalingMode=Treat bit field as an integer
  Extract Bits1 : simulink/Logic and Bit Operations/Extract Bits  bitsToExtract=Range of bits  numBits=8  bitIdxRange=[1]  outScalingMode=Treat bit field as an integer
  Vector Concatenate : Concatenate
  Out1 : Outport  VectorParamsAs1DForOutWhenUnconnected=off
  wires:
  In1/1 -> Extract Bits1/1, Extract Bits/1
  Extract Bits/1 -> Vector Concatenate/1
  Extract Bits1/1 -> Vector Concatenate/2
  Vector Concatenate/1 -> Data Type Conversion/1
  Data Type Conversion/1 -> Out1/1

== system RxTxFixedPointLibrary_noscopes/Receiver HDL/Frame Recover/Barker Locate/Measure Phase Ambiguity/Find Max and Set Output Shift ==
  In1 : Inport
  In2 : Inport  Port=2
  In4 : Inport  Port=3
  In5 : Inport  Port=4
  Enable : EnablePort
  Complex to Real-Imag{,1..3} (4 alike) : ComplexToRealImag  Output=Imag
  Direct Lookup Table (n-D)1 : LookupNDDirect  Commented=on  NumberOfTableDimensions=1  Table=-1i.*ones(1,4)  DiagnosticForOutOfRangeInput=Error  TableDataTypeStr=fixdt(1,16,13)
  Direct Lookup Table (n-D)2 : LookupNDDirect  NumberOfTableDimensions=1  Table=exp(-(0:pi/2:(pi*3/2)) .* 1i).'  DiagnosticForOutOfRangeInput=Error  TableDataTypeStr=fixdt(1,16,13)
  Maximum : dspstat3/Maximum  operation=maximum  fcn=Index  indexBase=Zero  operateOver=Each column  Dimension=1  InputProcessing=Columns as channels (frame based)  reset=None  roiEnable=off  roiType=Rectangles  roiPortion=Entire ROI  roiOutput=Individual statistics for each ROI  roiFlag=off  roundingMode=Floor  overflowMode=off  accumDataTypeStr=Inherit: Same as product output  accumLastDataTypeStr=Inherit: Same as product output
  Vector Concatenate : Concatenate  NumInputs=4
  Out1 : Outport  InitialOutput=0  VectorParamsAs1DForOutWhenUnconnected=off
  wires:
  Complex to Real-Imag/1 -> Vector Concatenate/1
  Complex to Real-Imag2/1 -> Vector Concatenate/3
  Complex to Real-Imag3/1 -> Vector Concatenate/4
  Complex to Real-Imag1/1 -> Vector Concatenate/2
  Vector Concatenate/1 -> Maximum/1
  Maximum/1 -> Direct Lookup Table (n-D)2/1
  In1/1 -> Complex to Real-Imag/1
  In5/1 -> Complex to Real-Imag3/1
  In2/1 -> Complex to Real-Imag1/1
  In4/1 -> Complex to Real-Imag2/1
  Direct Lookup Table (n-D)2/1 -> Out1/1

== system RxTxFixedPointLibrary_noscopes/Receiver HDL/Frame Recover/Barker Locate/Measure Phase Ambiguity/HDL Opt Complex FIR4 ==
  In1 : Inport
  validIn : Inport  Port=2
  Add : Sum  Inputs=+-  AccumDataTypeStr=fixdt(1,16,0)
  Complex to Real-Imag : ComplexToRealImag
  Discrete FIR Filter HDL Optimized : dsphdlfiltering/Discrete FIR Filter HDL Optimized  NumeratorSource=Property  Numerator=real(Taps)  NumeratorPrototype=[]  FilterStructure=Direct form systolic  SerializationOption=Minimum number of cycles between valid input samples  NumberOfCycles=2  NumberOfMultipliers=2  SimulateUsing=Code generation  roundingMode=Floor  overflowMode=off  CoefficientsDataTypeStr=Inherit: Same word length as input  CoefficientsMin=[]  CoefficientsMax=[]  OutputDataTypeStr=fixdt(1,16,0)  OutputMin=[]  OutputMax=[]  ResetInputPort=off  HDLGlobalReset=off
      settings: SourceProductBaseCode=DS
  Discrete FIR Filter HDL Optimized1 : dsphdlfiltering/Discrete FIR Filter HDL Optimized  NumeratorSource=Property  Numerator=imag(Taps)  NumeratorPrototype=[]  FilterStructure=Direct form systolic  SerializationOption=Minimum number of cycles between valid input samples  NumberOfCycles=2  NumberOfMultipliers=2  SimulateUsing=Code generation  roundingMode=Floor  overflowMode=off  CoefficientsDataTypeStr=Inherit: Same word length as input  CoefficientsMin=[]  CoefficientsMax=[]  OutputDataTypeStr=fixdt(1,16,0)  OutputMin=[]  OutputMax=[]  ResetInputPort=off  HDLGlobalReset=off
      settings: SourceProductBaseCode=DS
  Discrete FIR Filter HDL Optimized2 : dsphdlfiltering/Discrete FIR Filter HDL Optimized  NumeratorSource=Property  Numerator=real(Taps)  NumeratorPrototype=[]  FilterStructure=Direct form systolic  SerializationOption=Minimum number of cycles between valid input samples  NumberOfCycles=2  NumberOfMultipliers=2  SimulateUsing=Code generation  roundingMode=Floor  overflowMode=off  CoefficientsDataTypeStr=Inherit: Same word length as input  CoefficientsMin=[]  CoefficientsMax=[]  OutputDataTypeStr=fixdt(1,16,0)  OutputMin=[]  OutputMax=[]  ResetInputPort=off  HDLGlobalReset=off
      settings: SourceProductBaseCode=DS
  Discrete FIR Filter HDL Optimized3 : dsphdlfiltering/Discrete FIR Filter HDL Optimized  NumeratorSource=Property  Numerator=imag(Taps)  NumeratorPrototype=[]  FilterStructure=Direct form systolic  SerializationOption=Minimum number of cycles between valid input samples  NumberOfCycles=2  NumberOfMultipliers=2  SimulateUsing=Code generation  roundingMode=Floor  overflowMode=off  CoefficientsDataTypeStr=Inherit: Same word length as input  CoefficientsMin=[]  CoefficientsMax=[]  OutputDataTypeStr=fixdt(1,16,0)  OutputMin=[]  OutputMax=[]  ResetInputPort=off  HDLGlobalReset=off
      settings: SourceProductBaseCode=DS
  Logical Operator : Logic  Inputs=4  AllPortsSameDT=off  OutDataTypeStr=boolean
  Real-Imag to Complex : RealImagToComplex
  Subtract : Sum  OutDataTypeStr=int16
  Out1 : Outport  VectorParamsAs1DForOutWhenUnconnected=off
  validOut : Outport  Port=2  VectorParamsAs1DForOutWhenUnconnected=off
  wires:
  Add/1 -> Real-Imag to Complex/1
  Subtract/1 -> Real-Imag to Complex/2
  Real-Imag to Complex/1 -> Out1/1
  Discrete FIR Filter HDL Optimized3/1 -> Subtract/2
  Discrete FIR Filter HDL Optimized2/1 -> Subtract/1
  Complex to Real-Imag/2 -> Discrete FIR Filter HDL Optimized1/1, Discrete FIR Filter HDL Optimized2/1
  Discrete FIR Filter HDL Optimized3/2 -> Logical Operator/4
  Discrete FIR Filter HDL Optimized2/2 -> Logical Operator/3
  Complex to Real-Imag/1 -> Discrete FIR Filter HDL Optimized/1, Discrete FIR Filter HDL Optimized3/1
  In1/1 -> Complex to Real-Imag/1
  validIn/1 -> Discrete FIR Filter HDL Optimized/2, Discrete FIR Filter HDL Optimized1/2, Discrete FIR Filter HDL Optimized2/2, Discrete FIR Filter HDL Optimized3/2
  Discrete FIR Filter HDL Optimized1/1 -> Add/2
  Discrete FIR Filter HDL Optimized1/2 -> Logical Operator/2
  Discrete FIR Filter HDL Optimized/2 -> Logical Operator/1
  Logical Operator/1 -> validOut/1
  Discrete FIR Filter HDL Optimized/1 -> Add/1

== system RxTxFixedPointLibrary_noscopes/Receiver HDL/Frame Recover/Barker Locate/Measure Phase Ambiguity/HDL Opt Complex FIR5 ==
  In1 : Inport
  validIn : Inport  Port=2
  Add : Sum  Inputs=+-  AccumDataTypeStr=fixdt(1,16,0)
  Complex to Real-Imag : ComplexToRealImag
  Discrete FIR Filter HDL Optimized : dsphdlfiltering/Discrete FIR Filter HDL Optimized  NumeratorSource=Property  Numerator=real(Taps)  NumeratorPrototype=[]  FilterStructure=Direct form systolic  SerializationOption=Minimum number of cycles between valid input samples  NumberOfCycles=2  NumberOfMultipliers=2  SimulateUsing=Code generation  roundingMode=Floor  overflowMode=off  CoefficientsDataTypeStr=Inherit: Same word length as input  CoefficientsMin=[]  CoefficientsMax=[]  OutputDataTypeStr=fixdt(1,16,0)  OutputMin=[]  OutputMax=[]  ResetInputPort=off  HDLGlobalReset=off
      settings: SourceProductBaseCode=DS
  Discrete FIR Filter HDL Optimized1 : dsphdlfiltering/Discrete FIR Filter HDL Optimized  NumeratorSource=Property  Numerator=imag(Taps)  NumeratorPrototype=[]  FilterStructure=Direct form systolic  SerializationOption=Minimum number of cycles between valid input samples  NumberOfCycles=2  NumberOfMultipliers=2  SimulateUsing=Code generation  roundingMode=Floor  overflowMode=off  CoefficientsDataTypeStr=Inherit: Same word length as input  CoefficientsMin=[]  CoefficientsMax=[]  OutputDataTypeStr=fixdt(1,16,0)  OutputMin=[]  OutputMax=[]  ResetInputPort=off  HDLGlobalReset=off
      settings: SourceProductBaseCode=DS
  Discrete FIR Filter HDL Optimized2 : dsphdlfiltering/Discrete FIR Filter HDL Optimized  NumeratorSource=Property  Numerator=real(Taps)  NumeratorPrototype=[]  FilterStructure=Direct form systolic  SerializationOption=Minimum number of cycles between valid input samples  NumberOfCycles=2  NumberOfMultipliers=2  SimulateUsing=Code generation  roundingMode=Floor  overflowMode=off  CoefficientsDataTypeStr=Inherit: Same word length as input  CoefficientsMin=[]  CoefficientsMax=[]  OutputDataTypeStr=fixdt(1,16,0)  OutputMin=[]  OutputMax=[]  ResetInputPort=off  HDLGlobalReset=off
      settings: SourceProductBaseCode=DS
  Discrete FIR Filter HDL Optimized3 : dsphdlfiltering/Discrete FIR Filter HDL Optimized  NumeratorSource=Property  Numerator=imag(Taps)  NumeratorPrototype=[]  FilterStructure=Direct form systolic  SerializationOption=Minimum number of cycles between valid input samples  NumberOfCycles=2  NumberOfMultipliers=2  SimulateUsing=Code generation  roundingMode=Floor  overflowMode=off  CoefficientsDataTypeStr=Inherit: Same word length as input  CoefficientsMin=[]  CoefficientsMax=[]  OutputDataTypeStr=fixdt(1,16,0)  OutputMin=[]  OutputMax=[]  ResetInputPort=off  HDLGlobalReset=off
      settings: SourceProductBaseCode=DS
  Logical Operator : Logic  Inputs=4  AllPortsSameDT=off  OutDataTypeStr=boolean
  Real-Imag to Complex : RealImagToComplex
  Subtract : Sum  OutDataTypeStr=int16
  Out1 : Outport  VectorParamsAs1DForOutWhenUnconnected=off
  validOut : Outport  Port=2  VectorParamsAs1DForOutWhenUnconnected=off
  wires:
  Add/1 -> Real-Imag to Complex/1
  Subtract/1 -> Real-Imag to Complex/2
  Real-Imag to Complex/1 -> Out1/1
  Discrete FIR Filter HDL Optimized3/1 -> Subtract/2
  Discrete FIR Filter HDL Optimized2/1 -> Subtract/1
  Complex to Real-Imag/2 -> Discrete FIR Filter HDL Optimized1/1, Discrete FIR Filter HDL Optimized2/1
  Discrete FIR Filter HDL Optimized3/2 -> Logical Operator/4
  Discrete FIR Filter HDL Optimized2/2 -> Logical Operator/3
  Complex to Real-Imag/1 -> Discrete FIR Filter HDL Optimized/1, Discrete FIR Filter HDL Optimized3/1
  In1/1 -> Complex to Real-Imag/1
  validIn/1 -> Discrete FIR Filter HDL Optimized/2, Discrete FIR Filter HDL Optimized1/2, Discrete FIR Filter HDL Optimized2/2, Discrete FIR Filter HDL Optimized3/2
  Discrete FIR Filter HDL Optimized1/1 -> Add/2
  Discrete FIR Filter HDL Optimized1/2 -> Logical Operator/2
  Discrete FIR Filter HDL Optimized/2 -> Logical Operator/1
  Logical Operator/1 -> validOut/1
  Discrete FIR Filter HDL Optimized/1 -> Add/1

== system RxTxFixedPointLibrary_noscopes/Receiver HDL/Frame Recover/Barker Locate/Measure Phase Ambiguity/HDL Opt Complex FIR6 ==
  In1 : Inport
  validIn : Inport  Port=2
  Add : Sum  Inputs=+-  AccumDataTypeStr=fixdt(1,16,0)
  Complex to Real-Imag : ComplexToRealImag
  Discrete FIR Filter HDL Optimized : dsphdlfiltering/Discrete FIR Filter HDL Optimized  NumeratorSource=Property  Numerator=real(Taps)  NumeratorPrototype=[]  FilterStructure=Direct form systolic  SerializationOption=Minimum number of cycles between valid input samples  NumberOfCycles=2  NumberOfMultipliers=2  SimulateUsing=Code generation  roundingMode=Floor  overflowMode=off  CoefficientsDataTypeStr=Inherit: Same word length as input  CoefficientsMin=[]  CoefficientsMax=[]  OutputDataTypeStr=fixdt(1,16,0)  OutputMin=[]  OutputMax=[]  ResetInputPort=off  HDLGlobalReset=off
      settings: SourceProductBaseCode=DS
  Discrete FIR Filter HDL Optimized1 : dsphdlfiltering/Discrete FIR Filter HDL Optimized  NumeratorSource=Property  Numerator=imag(Taps)  NumeratorPrototype=[]  FilterStructure=Direct form systolic  SerializationOption=Minimum number of cycles between valid input samples  NumberOfCycles=2  NumberOfMultipliers=2  SimulateUsing=Code generation  roundingMode=Floor  overflowMode=off  CoefficientsDataTypeStr=Inherit: Same word length as input  CoefficientsMin=[]  CoefficientsMax=[]  OutputDataTypeStr=fixdt(1,16,0)  OutputMin=[]  OutputMax=[]  ResetInputPort=off  HDLGlobalReset=off
      settings: SourceProductBaseCode=DS
  Discrete FIR Filter HDL Optimized2 : dsphdlfiltering/Discrete FIR Filter HDL Optimized  NumeratorSource=Property  Numerator=real(Taps)  NumeratorPrototype=[]  FilterStructure=Direct form systolic  SerializationOption=Minimum number of cycles between valid input samples  NumberOfCycles=2  NumberOfMultipliers=2  SimulateUsing=Code generation  roundingMode=Floor  overflowMode=off  CoefficientsDataTypeStr=Inherit: Same word length as input  CoefficientsMin=[]  CoefficientsMax=[]  OutputDataTypeStr=fixdt(1,16,0)  OutputMin=[]  OutputMax=[]  ResetInputPort=off  HDLGlobalReset=off
      settings: SourceProductBaseCode=DS
  Discrete FIR Filter HDL Optimized3 : dsphdlfiltering/Discrete FIR Filter HDL Optimized  NumeratorSource=Property  Numerator=imag(Taps)  NumeratorPrototype=[]  FilterStructure=Direct form systolic  SerializationOption=Minimum number of cycles between valid input samples  NumberOfCycles=2  NumberOfMultipliers=2  SimulateUsing=Code generation  roundingMode=Floor  overflowMode=off  CoefficientsDataTypeStr=Inherit: Same word length as input  CoefficientsMin=[]  CoefficientsMax=[]  OutputDataTypeStr=fixdt(1,16,0)  OutputMin=[]  OutputMax=[]  ResetInputPort=off  HDLGlobalReset=off
      settings: SourceProductBaseCode=DS
  Logical Operator : Logic  Inputs=4  AllPortsSameDT=off  OutDataTypeStr=boolean
  Real-Imag to Complex : RealImagToComplex
  Subtract : Sum  OutDataTypeStr=int16
  Out1 : Outport  VectorParamsAs1DForOutWhenUnconnected=off
  validOut : Outport  Port=2  VectorParamsAs1DForOutWhenUnconnected=off
  wires:
  Add/1 -> Real-Imag to Complex/1
  Subtract/1 -> Real-Imag to Complex/2
  Real-Imag to Complex/1 -> Out1/1
  Discrete FIR Filter HDL Optimized3/1 -> Subtract/2
  Discrete FIR Filter HDL Optimized2/1 -> Subtract/1
  Complex to Real-Imag/2 -> Discrete FIR Filter HDL Optimized1/1, Discrete FIR Filter HDL Optimized2/1
  Discrete FIR Filter HDL Optimized3/2 -> Logical Operator/4
  Discrete FIR Filter HDL Optimized2/2 -> Logical Operator/3
  Complex to Real-Imag/1 -> Discrete FIR Filter HDL Optimized/1, Discrete FIR Filter HDL Optimized3/1
  In1/1 -> Complex to Real-Imag/1
  validIn/1 -> Discrete FIR Filter HDL Optimized/2, Discrete FIR Filter HDL Optimized1/2, Discrete FIR Filter HDL Optimized2/2, Discrete FIR Filter HDL Optimized3/2
  Discrete FIR Filter HDL Optimized1/1 -> Add/2
  Discrete FIR Filter HDL Optimized1/2 -> Logical Operator/2
  Discrete FIR Filter HDL Optimized/2 -> Logical Operator/1
  Logical Operator/1 -> validOut/1
  Discrete FIR Filter HDL Optimized/1 -> Add/1
